simulink model "uncontrolled1"  (R2014a)
settings: Solver=ode45  StartTime=0.0  StopTime=0.1  RelTol=1e-3
values from neighbouring files (symbols this model uses):
  f1 = b    [uncontrolled.m]
  l1 = d    [uncontrolled.m]
  r1 = c    [uncontrolled.m]
  v1 = a    [uncontrolled.m]
libraries: powerlib x9
settings Model: Creator=SAMBIT  LastModifiedBy=SAMBIT

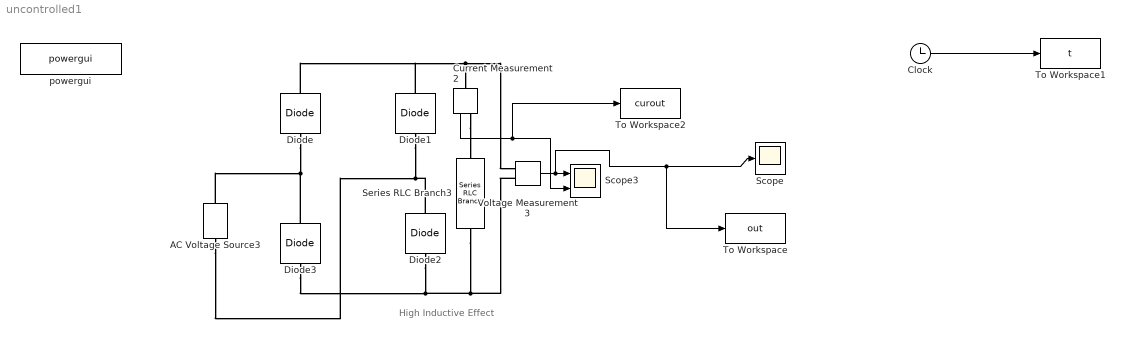
== system uncontrolled1 ==
  note: High Inductive Effect
  AC Voltage Source3 : powerlib/Electrical Sources/AC Voltage Source  Amplitude=v1  Phase=0  Frequency=f1  SampleTime=0  Measurements=None
  Clock : Clock
  Current Measurement2 : powerlib/Measurements/Current Measurement  PhasorSimulation=off  OutputType=Complex  PSBequivalent=0
  Diode{,1..3} (4 alike) : powerlib/Power Electronics/Diode  Ron=0.001  Lon=0  Vf=0.8  IC=0  UseSnubber=off  Rs=500  Cs=250e-9  Measurements=off
  Scope : Scope
  Scope3 : Scope  NumInputPorts=2
      settings: YMin=-5~-0.2  YMax=5~0.2  SaveName=SPBR_HL  MaxDataPoints=5000000  SampleInput=on  SampleTime=5e-6
  Series RLC Branch3 : powerlib/Elements/Series RLC Branch  LConnTagsString=__new0  RConnTagsString=__new0  BranchType=RL  Resistance=r1  Inductance=l1  SetiL0=off  InitialCurrent=0  Capacitance=1e-6  Setx0=off  InitialVoltage=0  Measurements=None
  To Workspace : ToWorkspace  VariableName=out  SampleTime=-1
  To Workspace1 : ToWorkspace  VariableName=t  SampleTime=-1
  To Workspace2 : ToWorkspace  VariableName=curout  SampleTime=-1
  Voltage Measurement3 : powerlib/Measurements/Voltage Measurement  PhasorSimulation=off  OutputType=Complex  PSBequivalent=0
  powergui : powerlib/powergui  Priority=1  SimulationMode=Discrete  SolverType=Tustin  SampleTime=5e-6  frequency=60  SPID=off  DisableSnubberDevices=off  DisableRonSwitches=off  DisableVfSwitches=off  SwTol=0  Interpol=off  DisplayEquations=off  Ts=0  methode=off  frequencyindice=60  Pbase=100e6  ErrMax=1e-4  Iterations=50  UnitsV=kV  UnitsW=MW  FunctionMessages=off  echomessages=off  HookPort=off  EnableUseOfTLC=off  x0status=blocks  RestoreLinks=warning  ResistiveCurrentMeasurement=off  Frange=[0:2:500]  Ylog=off  Xlog=on  ShowGrid=off  save=off  variable=ZData  structure=SPBR_R  ZoomFFT=off  StartTime=0.0  cycles=1  DisplayStyle=1  fundamental=100  FreqAxis=off  MaxFrequency=1000  frequencyindicesteady=1  RmsSteady=1  display=off
  wires:
  Current Measurement2/1 -> To Workspace2/1, Scope3/2
  Clock/1 -> To Workspace1/1
  Voltage Measurement3/1 -> To Workspace/1, Scope/1, Scope3/1
  connections:
  AC Voltage Source3/LConn1 -- Diode2/RConn1 -- Diode1/LConn1
  Voltage Measurement3/LConn2 -- Series RLC Branch3/RConn1 -- Diode3/LConn1 -- Diode2/LConn1
  AC Voltage Source3/RConn1 -- Diode3/RConn1 -- Diode/LConn1
  Diode/RConn1 -- Diode1/RConn1 -- Current Measurement2/LConn1 -- Voltage Measurement3/LConn1
  Current Measurement2/RConn1 -- Series RLC Branch3/LConn1
